simulink model "playback_data"  (R2015a)
settings: Solver=FixedStepDiscrete  SolverMode=SingleTasking  StartTime=76  StopTime=110  FixedStep=sample_time  RelTol=1e-3
undefined symbols (not defined in the file): A1_notch_f1, A2_notch_f1, A_kalman_swing_load, A_kalman_transverse, A_kalman_vertical, A_lpf_accelerometer, A_lpf_dtau, A_lpf_fourbar_angles, A_lpf_imu, A_lpf_lateral_angle, B1_lpf_accelerometer, B1_lpf_dtau, B1_lpf_fourbar_angles, B1_lpf_imu, B1_lpf_lateral_angle, B1_notch_f1, B2_lpf_accelerometer, B2_lpf_dtau, B2_lpf_fourbar_angles, B2_lpf_imu, B2_lpf_lateral_angle, B2_notch_f1, B_dx_versus_x0, B_kalman_swing_load, B_kalman_transverse, B_kalman_vertical, backwards_K_sag_of_t, backwards_P_sag_of_t, C_kalman_swing_load, C_kalman_transverse, C_kalman_vertical, com_leg_motor, com_torso, contact_threshold, control_start_time, d_ankle_to_foot, d_vertical_com, desired_com_forward_velocity, desired_com_lateral_velocity, desired_initial_leg_roll_left, desired_initial_leg_roll_right, desired_stance_beta2, desired_standing_torso_pitch, desired_standing_torso_roll, desired_standing_z, desired_torso_pitch, desired_torso_roll, Discrete, enable_bouncing, fcut_contact, fdesignblkfcn, forward_dx_of_dxstar, forward_x_of_dxstar, g, gcbh, HIP_MTR_MAX_CONT_TORQUE, HIP_MTR_MAX_TORQUE, i_leg_motor, i_robot, i_torso ... (+78)
libraries: simulink x65, dsparch4 x18, ctrlSharedLib x14, dspfdesign x4
(part 2 of 13)

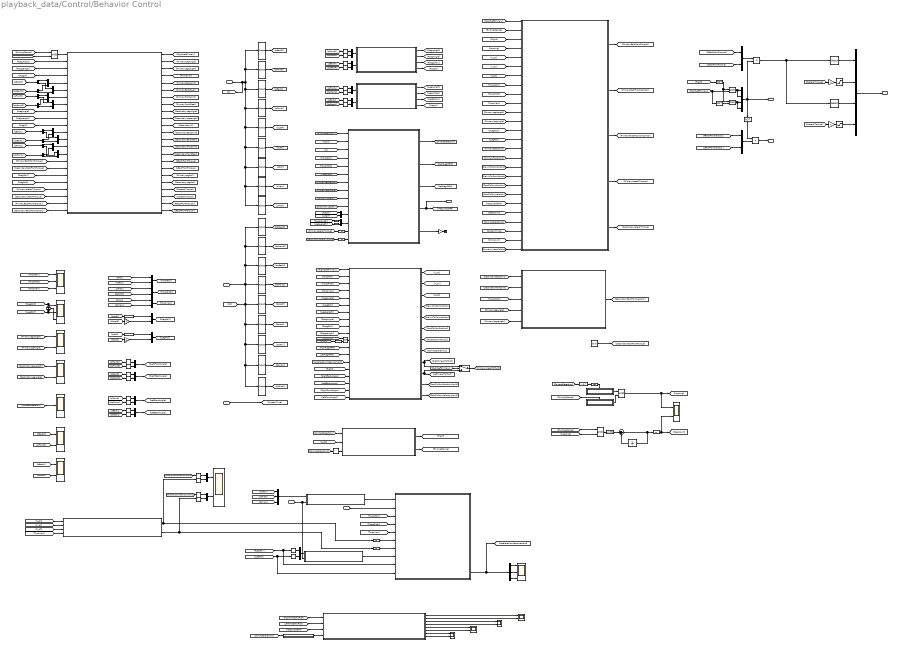
== system playback_data/Control/Behavior Control ==
  note: Signal Routing
  note: Begin Control
  note: Position & Velocity Estimation
  note: Force Estimation
  note: Leg/Spring Measurements
  note: Torque Commands
  note: Secondary Leg Behavior
  note: Primary Leg + Lateral Behavior
  note: Inputs
  note: q Order:
      |
      | backJointR
      | backGearR
      | frontJointR
      | frontGearR
      |
      | backJointL
      | backGearL
      | frontJointL
      | frontGearL
      |
      | latR
      | latL
      |
      | torsoRoll
      | torsoYaw
      | torsoPitch
  note: Motor Order:
      |
      | backR
      | frontR
      | latR
      | backL
      | frontL
      | latL
  note: Angle Conversions
  note: Contact Estimation
  note: Logging
  note: Acceleration Measurement
  note: Knee Torque Estimation
  Enabled [true/false] : Inport
  Body XYZ Acceleration [m/s^2] x3 : Inport  Port=2
  dq : Inport  Port=3
  q : Inport  Port=4
  time : Inport  Port=5
  At Least One Stance Detected : Subsystem
  COM Acceleration Measurement : Scope  NumInputPorts=3
      settings: YMin=-10~-12.5~-15  YMax=7.5~7.5~15  SaveName=ScopeData34  SampleInput=on
  COM World Frame X : Scope  NumInputPorts=2
      settings: TimeRange=3.175000000000004  YMin=-0.004~-0.175  YMax=0.02~0.225  SaveName=ScopeData35  SampleInput=on
  Compare To Constant : simulink/Logic and Bit Operations/Compare To Constant  relop=>  const=0.7  OutDataTypeStr=boolean
  Compute COM Translational Acceleration (IMU uses non-rotating measurement frame) : MATLAB Function  TreatAsAtomicUnit=on
  Compute Forces1 : Subsystem
  Compute World Frame COM Coordinates from Yawed Frame : MATLAB Function  TreatAsAtomicUnit=on
  Constant : Constant  Value=[0 0]
  Contact : Scope
      settings: YMin=0.3  YMax=0.9  SaveName=ScopeData11  SampleInput=on
  Contact State Machine : Subsystem
  Data Type Conversion : DataTypeConversion  OutDataTypeStr=uint32
  Demux : Demux  Outputs=3
  Demux{3..10} (8 alike) : Demux  Outputs=2
  Estimate Angular Accelerations2 : Subsystem
  Estimate Angular Accelerations3 : Subsystem
  Exited Stance : Subsystem
  Force Estimation : Subsystem
  Gain{1..2,12..13} (4 alike) : Gain  Gain=-1
  Hopping / Steps : Scope  NumInputPorts=2
      settings: YMin=1~1  YMax=1~1  SaveName=ScopeData33  SampleInput=on
  Knee Torques : MATLAB Function  TreatAsAtomicUnit=on
  L Knee Torques from Accelerometer : Scope  NumInputPorts=2
      settings: YMin=-1000~-1250  YMax=1500~2000  SaveName=ScopeData42  SampleInput=on
  L Knee Torques from Forward Dynamics : Scope  NumInputPorts=2
      settings: YMin=-75~-220  YMax=250~0  SaveName=ScopeData43  SampleInput=on
  L Leg Calculator : Subsystem
  Left Lateral Torque Saturation : Saturate  UpperLimit=max_torque_lateral  LowerLimit=-max_torque_lateral
      settings: AttributesFormatString=Top: %<UpperLimit>\nBottom: %<LowerLimit>
  Left Leg Fourbar Positions : Scope  NumInputPorts=2
      settings: YMin=4.05~2.275  YMax=4.17~2.375  SaveName=ScopeData17  SampleInput=on
  Logical Operator : Logic  IconShape=distinctive  AllPortsSameDT=off  OutDataTypeStr=boolean
  Logical Operator{1,3,5,7} (4 alike) : Logic  AllPortsSameDT=off  OutDataTypeStr=boolean
  Logical Operator2 : Logic  Operator=OR  AllPortsSameDT=off  OutDataTypeStr=boolean
  Logical Operator{4,6,8..9} (4 alike) : Logic  Operator=NOT  AllPortsSameDT=off  OutDataTypeStr=boolean
  Mux : Mux
  Mux{1..2,4..24,26..27,30..31,33} (28 alike) : Mux  Inputs=2
  Mux28 : Mux  Inputs=3
  Mux3 : Mux
  Primary Leg Length / Angle : Scope  NumInputPorts=2
      settings: YMin=0.3~0  YMax=0.9~3.5  SaveName=ScopeData21  SampleInput=on
  Primary Secondary Leg Swap : Subsystem
  Primary and Lateral Behavior : Subsystem
  Product : Product
  Product1 : Product
  R Knee Torques from Accelerometer : Scope  NumInputPorts=2
      settings: YMin=0.95~0.95  YMax=1.05~1.05  SaveName=ScopeData41  SampleInput=on
  R Knee Torques from Forward Dynamics : Scope  NumInputPorts=2
      settings: YMin=0.95~0.95  YMax=1.05~1.05  SaveName=ScopeData40  SampleInput=on
  R Leg Calculator : Subsystem
  Right Lateral Torque Saturation : Saturate  UpperLimit=max_torque_lateral  LowerLimit=-max_torque_lateral
      settings: AttributesFormatString=Top: %<UpperLimit>\nBottom: %<LowerLimit>
  Right Left Symmetry Leg Roll : Scope  NumInputPorts=3
      settings: YMin=-0.2~-0.5~-0.5  YMax=1.3~1.8~0.5  SaveName=ScopeData19  SampleInput=on
  Right Leg Fourbar Positions : Scope  NumInputPorts=2
      settings: YMin=3.19015~1.00606  YMax=3.99645~2.79375  SaveName=ScopeData16
  Roll Pitch Yaw : Scope  NumInputPorts=3
      settings: YMin=-1000~-5~-5  YMax=1000~5~5  SampleInput=on
  Secondary Leg Behavior : Subsystem
  Secondary Leg Length / Angle : Scope  NumInputPorts=2
      settings: YMin=-1~-0.8  YMax=1~1.4  SaveName=ScopeData22  SampleInput=on
  Selector : Selector  InputPortWidth=4  Indices=[1 2]
  Selector1 : Selector  InputPortWidth=13  Indices=[10]
  Selector10 : Selector  InputPortWidth=13  Indices=[7 8]
  Selector11 : Selector  InputPortWidth=13  Indices=[9]
  Selector12 : Selector  InputPortWidth=13  Indices=[1 2]
  Selector13 : Selector  InputPortWidth=13  Indices=[3 4]
  Selector{14..17,19,24..27,29..37} (18 alike) : Selector  InputPortWidth=2  Indices=[1]
  Selector18 : Selector  InputPortWidth=13  Indices=[13]
  Selector2 : Selector  InputPortWidth=13  Indices=[5 6]
  Selector20 : Selector  InputPortWidth=13  Indices=[13]
  Selector21 : Selector  InputPortWidth=13  Indices=[11]
  Selector22 : Selector  InputPortWidth=13  Indices=[12]
  Selector23 : Selector  InputPortWidth=13  Indices=[11]
  Selector28 : Selector  InputPortWidth=13  Indices=[12]
  Selector3 : Selector  InputPortWidth=4  Indices=[3 4]
  Selector38 : Selector  InputPortWidth=3  Indices=[3]
  Selector4 : Selector  InputPortWidth=13  Indices=[7 8]
  Selector41 : Selector  InputPortWidth=2  Indices=[2]
  Selector42 : Selector  InputPortWidth=2  Indices=[2]
  Selector{43..46} (4 alike) : Selector  InputPortWidth=3  Indices=[1]
  Selector5 : Selector  InputPortWidth=13  Indices=[9]
  Selector6 : Selector  InputPortWidth=13  Indices=[1 2]
  Selector7 : Selector  InputPortWidth=13  Indices=[3 4]
  Selector8 : Selector  InputPortWidth=13  Indices=[10]
  Selector9 : Selector  InputPortWidth=13  Indices=[5 6]
  State Estimation : Subsystem
  Sum1 : Sum  Inputs=|++  OutMin=0
  Sum3 : Sum  Inputs=-|+
  Switch : Switch  Criteria=u2 ~= 0
  Terminator6 : Terminator
  Unit Delay : UnitDelay  SampleTime=-1
  Unit Delay{1..6} (6 alike) : UnitDelay  SampleTime=sample_time
  lateral_coordinates : Fcn  Expr=pi/2-u
  lateral_coordinates1 : Fcn  Expr=pi/2-u
  torso_roll_acceleration : Gain
  Torque Commands [Nm] x6 : Outport  OutputWhenDisabled=reset  InitialOutput=[0 0 0 0 0 0]
  Velocity Commands [rad/s] x4 : Outport  Port=2  OutputWhenDisabled=reset  InitialOutput=[0 0 0 0 0 0]
  Stance / Swing Control [1/0] x4 : Outport  Port=3  OutputWhenDisabled=reset  InitialOutput=[0 0 0 0 0 0]
  GRF XYZ estimates [N N N] : Outport  Port=4  OutputWhenDisabled=reset  InitialOutput=[0 0 0 0 0 0]
  wires:
  Selector46/1 -> Mux33/1
  Selector45/1 -> Mux31/1
  Selector44/1 -> Mux31/2
  Selector43/1 -> Mux33/2
  [FootToComPositionWorld] -> Selector46/1
  [FootToComVelocityWorld] -> Selector45/1
  Mux31/1 -> COM World Frame X/2
  Mux33/1 -> COM World Frame X/1
  [TorsoYaw] -> Compute World Frame COM Coordinates from Yawed Frame/4(torso_yaw)
  [Z_dZ] -> Compute World Frame COM Coordinates from Yawed Frame/3(Z_dZ)
  [Y_dY] -> Compute World Frame COM Coordinates from Yawed Frame/2(Y_dY)
  [X_dX] -> Compute World Frame COM Coordinates from Yawed Frame/1(X_dX)
  Compute World Frame COM Coordinates from Yawed Frame/1(com_position_world) -> Selector43/1, Unit Delay5/1
  Compute World Frame COM Coordinates from Yawed Frame/2(com_velocity_world) -> Selector44/1, Unit Delay6/1
  Unit Delay6/1 -> Compute COM Translational Acceleration (IMU uses non-rotating measurement frame)/7(com_velocity_world)
  Unit Delay5/1 -> Compute COM Translational Acceleration (IMU uses non-rotating measurement frame)/6(com_position_world)
  [TorsoYaw] -> Compute COM Translational Acceleration (IMU uses non-rotating measurement frame)/5(torso_yaw)
  Estimate Angular Accelerations3/1(Angular Accelerations [rad/s^2] x2) -> Compute COM Translational Acceleration (IMU uses non-rotating measurement frame)/8(hip_roll_accelerations)
  Mux30/1 -> Estimate Angular Accelerations3/1(Angular Velocities [rad/s] x2)
  Selector42/1 -> Mux30/2
  Selector41/1 -> Mux30/1
  [LLegRoll] -> Compute COM Translational Acceleration (IMU uses non-rotating measurement frame)/10(left_hip_roll), Selector42/1
  [RLegRoll] -> Compute COM Translational Acceleration (IMU uses non-rotating measurement frame)/9(right_hip_roll), Selector41/1
  Estimate Angular Accelerations2/1(Angular Accelerations [rad/s^2] x3) -> Compute COM Translational Acceleration (IMU uses non-rotating measurement frame)/1(torso_angular_accelerations)
  Body XYZ Acceleration [m/s^2] x3/1 -> Compute COM Translational Acceleration (IMU uses non-rotating measurement frame)/2(imu_translational_accelerations_body)
  Enabled [true/false]/1 -> Estimate Angular Accelerations3/2(Enabled), Estimate Angular Accelerations2/2(Enabled)
  Mux28/1 -> Estimate Angular Accelerations2/1(Angular Velocities [rad/s] x3)
  [dqYaw] -> Mux28/3
  [dqPitch] -> Mux28/2
  [dqRoll] -> Mux28/1
  [TorsoRoll] -> Compute COM Translational Acceleration (IMU uses non-rotating measurement frame)/3(torso_roll)
  [TorsoPitch] -> Compute COM Translational Acceleration (IMU uses non-rotating measurement frame)/4(torso_pitch)
  Demux/3 -> COM Acceleration Measurement/3
  Demux/1 -> COM Acceleration Measurement/1
  Demux/2 -> COM Acceleration Measurement/2
  Compute COM Translational Acceleration (IMU uses non-rotating measurement frame)/6(com_acceleration_yawed) -> [AccelerationMeasurement], Demux/1
  Switch/1 -> [PrimaryKneesToFoot]
  [RightLeftPrimary] -> Switch/2
  [LeftFrontAngle] -> State Estimation/19(Left Front [rad rad/s])
  [RightFrontAngle] -> State Estimation/18(Right Front [rad rad/s])
  [LeftBackAngle] -> State Estimation/17(Left Back [rad rad/s])
  [RightBackAngle] -> State Estimation/16(Right Back [rad rad/s])
  State Estimation/10(Left Knees to Foot [m m m] x2) -> [LeftKneesToFoot], Switch/3
  State Estimation/9(Right Knees to Foot [m m m] x2) -> Switch/1, [RightKneesToFoot]
  State Estimation/8(COM Acceleration [m/s^2] x3) -> [ComAccelerations]
  [AccelerationMeasurement] -> State Estimation/14(" Acceleration Measurement [m/s^2] x3")
  State Estimation/1("Horizontal COM [m, m/s]") -> [X_dX]
  State Estimation/3("Vertical COM [m, m/s]") -> [Z_dZ]
  [RLegLength] -> State Estimation/10(Right Leg Length [m m/s])
  [TorsoRoll] -> State Estimation/2(Torso Roll [rad rad/s])
  [TorsoPitch] -> State Estimation/3(Torso Pitch [rad rad/s])
  [RLegRoll] -> State Estimation/9(Right Leg Roll [rad rad/s])
  [LLegRoll] -> State Estimation/6(Left Leg Roll [rad rad/s])
  [LLegLength] -> State Estimation/7(Left Leg Length [m m/s])
  [LLegAngle] -> State Estimation/5(Left Leg Sagittal Angle [rad rad/s])
  [RLegAngle] -> State Estimation/8(Right Leg Sagittal Angle [rad rad/s])
  [RightLeftPrimary] -> State Estimation/1(Right or Left [1/0])
  Logical Operator2/1 -> State Estimation/11(Enable Kalman Filtering [1/0])
  [RightLegGRFs] -> State Estimation/12(Right GRF [X Y Z] [N N N])
  [LeftLegGRFs] -> State Estimation/13(Left GRF [X Y Z] [N N N])
  State Estimation/4(Pelvis to COM Position [m m m]) -> [PelvisToComPosition]
  State Estimation/5(Pelvis to COM Velocity [m/s m/s m/s]) -> [PelvisToComVelocity]
  State Estimation/2("Lateral COM [m, m/s]") -> [Y_dY]
  [TorsoYaw] -> State Estimation/4(Torso Yaw [rad rad/s])
  State Estimation/6(Foot to COM Position [m m m]) -> [FootToComPosition]
  State Estimation/7(Foot to COM Velocity [m/s m/s m/s]) -> [FootToComVelocity]
  [hopping] -> Logical Operator2/1
  Logical Operator4/1 -> Logical Operator2/2
  [flight] -> Logical Operator4/1
  [flight] -> State Estimation/15(Flight [1/0])
  State Estimation/11(COM Position World [m m m]) -> [FootToComPositionWorld]
  State Estimation/12(COM Velocity World [m/s m/s m/s]) -> [FootToComVelocityWorld]
  [ExitingStance] -> Exited Stance/Enable
  Data Type Conversion/1 -> Sum1/1
  Logical Operator1/1 -> Data Type Conversion/1
  Sum1/1 -> Unit Delay/1, Unit Delay2/1
  Unit Delay/1 -> Sum1/2
  [RLateralTorque] -> Gain2/1
  [SecondaryBackJoint] -> Secondary Leg Behavior/1(Secondary Back Load [rad rad/s])
  [SecondaryFrontJoint] -> Secondary Leg Behavior/2(Secondary Front Load [rad rad/s])
  Primary and Lateral Behavior/3(Primary Force or Position Control [1/0]) -> [PrimaryForcePositionControl]
  Primary and Lateral Behavior/1(Primary Back/Front SEA Torques [Nm] x2) -> [PrimaryBackFrontTorque]
  Primary Secondary Leg Swap/1(Right/Left Primary [1/0]) -> [RightLeftPrimary]
  Logical Operator/1 -> Primary Secondary Leg Swap/1(Exiting Stance [1/0])
  Primary Secondary Leg Swap/17(L Back/Front SEA Torque [Nm Nm]) -> [LBackFrontTorque]
  Primary Secondary Leg Swap/16(R Back/Front SEA Torque [Nm Nm]) -> [RBackFrontTorque]
  Primary Secondary Leg Swap/11(Secondary Leg w [m]) -> [SecondaryW]
  Primary Secondary Leg Swap/15(Secondary Front Gear [rad rad/s]) -> [SecondaryFrontGear]
  Primary Secondary Leg Swap/14(Secondary Front Joint [rad rad/s]) -> [SecondaryFrontJoint]
  Primary Secondary Leg Swap/13(Secondary Back Gear [rad rad/s]) -> [SecondaryBackGear]
  Primary Secondary Leg Swap/12(Secondary Back Joint [rad rad/s]) -> [SecondaryBackJoint]
  Primary Secondary Leg Swap/8(Primary Front Gear [rad rad/s]) -> [PrimaryFrontGear]
  Primary Secondary Leg Swap/7(Primary Front Joint [rad rad/s]) -> [PrimaryFrontJoint]
  Primary Secondary Leg Swap/6(Primary Back Gear [rad rad/s]) -> [PrimaryBackGear]
  Primary Secondary Leg Swap/5(Primary Back Joint [rad rad/s]) -> [PrimaryBackJoint]
  [SecondaryBackFrontTorque] -> Primary Secondary Leg Swap/17(Secondary Back/Front SEA Torque [Nm Nm])
  [PrimaryBackFrontTorque] -> Primary Secondary Leg Swap/16(Primary Back/Front SEA Torque [Nm Nm])
  Demux9/2 -> Mux13/2
  Demux9/1 -> Mux16/2
  Demux10/2 -> Mux13/1
  Demux10/1 -> Mux16/1
  [qBackL] -> Demux10/1
  [dqBackL] -> Demux9/1
  Demux8/2 -> Mux15/2
  Demux8/1 -> Mux14/2
  Demux7/2 -> Mux15/1
  Demux7/1 -> Mux14/1
  Mux15/1 -> Primary Secondary Leg Swap/15(L Front Gear [rad rad/s])
  Mux14/1 -> Primary Secondary Leg Swap/14(L Front Joint [rad rad/s])
  Mux13/1 -> Primary Secondary Leg Swap/13(L Back Gear [rad rad/s])
  Mux16/1 -> Primary Secondary Leg Swap/12(L Back Joint [rad rad/s])
  [dqFrontL] -> Demux8/1
  [qFrontL] -> Demux7/1
  Demux5/2 -> Mux10/2
  Demux5/1 -> Mux9/2
  Demux6/2 -> Mux10/1
  Demux6/1 -> Mux9/1
  [qBackR] -> Demux6/1
  [dqBackR] -> Demux5/1
  Demux4/2 -> Mux12/2
  Demux4/1 -> Mux11/2
  Demux3/2 -> Mux12/1
  Demux3/1 -> Mux11/1
  Mux12/1 -> Primary Secondary Leg Swap/8(R Front Gear [rad rad/s])
  Mux11/1 -> Primary Secondary Leg Swap/7(R Front Joint [rad rad/s])
  Mux10/1 -> Primary Secondary Leg Swap/6(R Back Gear [rad rad/s])
  Mux9/1 -> Primary Secondary Leg Swap/5(R Back Joint [rad rad/s])
  [dqFrontR] -> Demux4/1
  [qFrontR] -> Demux3/1
  Primary Secondary Leg Swap/9(Secondary Leg Angle [rad rad/s]) -> [SecondaryLegAngle]
  Primary Secondary Leg Swap/10(Secondary Leg Length [rad rad/s]) -> [SecondaryLegLength]
  [LLegW] -> Primary Secondary Leg Swap/11(L Leg w [m])
  [LLegLength] -> Primary Secondary Leg Swap/10(L Leg Length [m m/s])
  [LLegAngle] -> Primary Secondary Leg Swap/9(L Leg Angle [rad rad/s])
  [RLegW] -> Primary Secondary Leg Swap/4(R Leg w [m])
  [RLegLength] -> Primary Secondary Leg Swap/3(R Leg Length [m m/s])
  [RLegAngle] -> Primary Secondary Leg Swap/2(R Leg Angle [rad rad/s])
  Primary Secondary Leg Swap/3(Primary Leg Length [m m/s]) -> [PrimaryLegLength]
  Primary Secondary Leg Swap/4(Primary Leg w [m]) -> [PrimaryW]
  Primary Secondary Leg Swap/2(Primary Leg Angle [rad rad/s]) -> [PrimaryLegAngle]
  [TorsoPitch] -> Secondary Leg Behavior/3(Torso Pitch [rad rad/s])
  L Leg Calculator/4(w [m]) -> [LLegW]
  R Leg Calculator/4(w [m]) -> [RLegW]
  Selector26/1 -> Mux4/1
  Selector27/1 -> Mux4/2
  Selector25/1 -> Mux5/2
  Selector24/1 -> Mux5/1
  L Leg Calculator/3(Leg Splay [rad rad/s]) -> [LLegSplay]
  L Leg Calculator/2(Leg Angle [rad rad/s]) -> [LLegAngle]
  L Leg Calculator/1("Leg Length [m m/s] ") -> [LLegLength]
  Mux4/1 -> L Leg Calculator/2(Back [rad rad/s])
  Mux5/1 -> L Leg Calculator/1(Front [rad rad/s])
  [dqFrontL] -> Selector25/1
  [qFrontL] -> Selector24/1
  [dqBackL] -> Selector27/1
  [qBackL] -> Selector26/1
  Selector23/1 -> [qRoll]
  Selector18/1 -> [qPitch]
  q/1 -> [q], Selector1/1, Selector23/1, Selector28/1, Selector18/1, Selector5/1, Selector4/1, Selector2/1, Selector7/1, Selector6/1
  Selector16/1 -> Mux1/1
  Selector17/1 -> Mux1/2
  Selector15/1 -> Mux2/2
  Selector14/1 -> Mux2/1
  R Leg Calculator/3(Leg Splay [rad rad/s]) -> [RLegSplay]
  R Leg Calculator/2(Leg Angle [rad rad/s]) -> [RLegAngle]
  R Leg Calculator/1("Leg Length [m m/s] ") -> [RLegLength]
  Mux1/1 -> R Leg Calculator/2(Back [rad rad/s])
  Mux2/1 -> R Leg Calculator/1(Front [rad rad/s])
  [dqFrontR] -> Selector15/1
  [qFrontR] -> Selector14/1
  [dqBackR] -> Selector17/1
  [qBackR] -> Selector16/1
  Selector5/1 -> [qLatR]
  Selector1/1 -> [qLatL]
  Selector6/1 -> [qBackR]
  Selector7/1 -> [qFrontR]
  Selector2/1 -> [qBackL]
  Selector4/1 -> [qFrontL]
  [PrimaryLegAngle] -> Secondary Leg Behavior/4(Primary Leg Angle [rad rad/s])
  [PrimaryLegLength] -> Secondary Leg Behavior/5(Primary Leg Length [m m/s])
  Selector28/1 -> [qYaw]
  Force Estimation/1(Leg Plane Force for Contact Detection [body weight]) -> [ContactDetection]
  Force Estimation/2(Right GRF [X Y Z] [N N N]) -> [RightLegGRFs]
  [LLateralTorque] -> Gain1/1
  Force Estimation/3(Left GRF [X Y Z] [N N N]) -> [LeftLegGRFs]
  Force Estimation/4(GRF XYZ estimates [N N N]) -> GRF XYZ estimates [N N N]/1, [MeasuredGRF]
  Primary Secondary Leg Swap/18("Primary Leg Roll [rad, rad/s]") -> [PrimaryLegRoll]
  Primary Secondary Leg Swap/19("Secondary Leg Roll [rad, rad/s]") -> [SecondaryLegRoll]
  [RLegRoll] -> Primary Secondary Leg Swap/18("Right Leg Roll [rad, rad/s]")
  [LLegRoll] -> Primary Secondary Leg Swap/19("Left Leg Roll [rad, rad/s]")
  Unit Delay2/1 -> Hopping / Steps/2, [StepCount]
  [ExitingStance] -> Logical Operator1/1
  [hopping] -> Logical Operator1/2
  [hopping] -> Logical Operator/2
  [ExitingStance] -> Logical Operator/1
  [RightLeftPrimary] -> Force Estimation/1(Right/Left Primary)
  [flight] -> Force Estimation/2(Flight [1/0])
  [TorsoRoll] -> Force Estimation/4(Torso Roll [rad rad/s])
  [TorsoYaw] -> Force Estimation/6(Torso Yaw [rad rad/s])
  [TorsoPitch] -> Force Estimation/5(Torso Pitch [rad rad/s])
  [q] -> Force Estimation/3(q)
  [PrimaryLegLength] -> Force Estimation/7(Primary Leg Length [m m/s])
  [PrimaryLegAngle] -> Force Estimation/8(Primary Leg Angle [rad rad/s])
  [PrimaryLegRoll] -> Force Estimation/9(Primary Leg Roll [rad rad/s])
  [RLegW] -> Mux19/1
  [LLegW] -> Mux19/2
  Mux19/1 -> Force Estimation/11(Leg Width Right/Left [m m])
  [RLegLength] -> Selector19/1
  Mux20/1 -> Force Estimation/12(Leg Length Right/Left [m m])
  [SecondaryLegRoll] -> Force Estimation/10(Secondary Leg Roll [rad rad/s])
  [PrimaryLateralTorque] -> Unit Delay3/1
  [SecondaryLateralTorque] -> Unit Delay4/1
  torso_roll_acceleration/1 -> Terminator6/1
  Force Estimation/5(Torso Roll Acceleration [rad/s^2]) -> torso_roll_acceleration/1
  [PrimaryLateralTorque] -> Primary Secondary Leg Swap/20(Primary Lateral Torque [Nm])
  [SecondaryLateralTorque] -> Primary Secondary Leg Swap/21(Secondary Lateral Torque [Nm])
  Primary Secondary Leg Swap/20(Right Lateral Torque [Nm]) -> [RLateralTorque]
  Primary Secondary Leg Swap/21(Left Lateral Torque [Nm]) -> [LLateralTorque]
  Right Lateral Torque Saturation/1 -> Mux/2
  Left Lateral Torque Saturation/1 -> Mux/4
  Primary and Lateral Behavior/5(Secondary Lateral Torque [Nm]) -> [SecondaryLateralTorque]
  Primary and Lateral Behavior/4(Primary Lateral Torque [Nm]) -> [PrimaryLateralTorque]
  Selector19/1 -> Mux20/1
  [LLegLength] -> Selector29/1
  Selector29/1 -> Mux20/2
  Unit Delay3/1 -> Force Estimation/13(Primary Lateral Torque [Nm])
  Unit Delay4/1 -> Force Estimation/14(Secondary Lateral Torque [Nm])
  Logical Operator3/1 -> Hopping / Steps/1, [hopping]
  Gain2/1 -> Right Lateral Torque Saturation/1
  Gain1/1 -> Left Lateral Torque Saturation/1
  [TorsoYaw] -> Primary and Lateral Behavior/10(Torso Yaw [rad rad/s])
  [LLegRoll] -> Primary and Lateral Behavior/14(Left Leg Roll [rad rad/s])
  [RLegRoll] -> Primary and Lateral Behavior/13(Right Leg Roll [rad rad/s])
  [Y_dY] -> Primary and Lateral Behavior/6("[y,  dy] [m, m/s]")
  [StepCount] -> Primary and Lateral Behavior/22(Steps Taken)
  [MeasuredGRF] -> Primary and Lateral Behavior/21(Measured GRF [N N N])
  [TorsoRoll] -> Primary and Lateral Behavior/8(Torso Roll [rad rad/s])
  [Z_dZ] -> Primary and Lateral Behavior/7("[z, dz] [m, m/s]")
  [X_dX] -> Primary and Lateral Behavior/5("[x, dx] [m, m/s]")
  [PelvisToComVelocity] -> Primary and Lateral Behavior/18(Pelvis to COM Velocity [m m m])
  [PelvisToComPosition] -> Primary and Lateral Behavior/17(Pelvis to COM Position [m m m])
  [TorsoPitch] -> Primary and Lateral Behavior/9(Torso Pitch [rad rad/s])
  [PrimaryFrontJoint] -> Primary and Lateral Behavior/16(Primary Front Load [rad rad/s])
  [PrimaryLegLength] -> Primary and Lateral Behavior/11(Leg Length [m m/s])
  [hopping] -> Primary and Lateral Behavior/4(Hopping [1/0])
  [RightLeftPrimary] -> Primary and Lateral Behavior/1(Right/Left [1/0])
  [PrimaryBackJoint] -> Primary and Lateral Behavior/15(Primary Back Load [rad rad/s])
  [PrimaryLegAngle] -> Primary and Lateral Behavior/12(Leg Angle [rad rad/s])
  Contact State Machine/1(flight [1/0]) -> [flight]
  [FootToComVelocity] -> Primary and Lateral Behavior/20(Foot to COM Velocity [m m m])
  [FootToComPosition] -> Primary and Lateral Behavior/19(Foot to COM Position [m m m])
  Contact State Machine/2(Exiting Stance [1/0]) -> [ExitingStance]
  [flight] -> Primary and Lateral Behavior/3(Flight [1/0])
  [ContactDetection] -> Contact State Machine/1(Contact Factor [body weight])
  [Z_dZ] -> Contact State Machine/2("[Z dZ] [m m/s]")
  [ExitingStance] -> Primary and Lateral Behavior/2(Exiting Stance [1/0])
  [TorsoYaw] -> Roll Pitch Yaw/3
  [TorsoPitch] -> Roll Pitch Yaw/2
  [TorsoRoll] -> Roll Pitch Yaw/1
  [LLegRoll] -> Sum3/2, Right Left Symmetry Leg Roll/2
  [RLegRoll] -> Sum3/1, Right Left Symmetry Leg Roll/1
  Sum3/1 -> Right Left Symmetry Leg Roll/3
  [PrimaryLegLength] -> Primary Leg Length / Angle/1
  [PrimaryLegAngle] -> Primary Leg Length / Angle/2
  [SecondaryLegLength] -> Secondary Leg Length / Angle/1
  [SecondaryLegAngle] -> Secondary Leg Length / Angle/2
  [ContactDetection] -> Contact/1
  Secondary Leg Behavior/1(Secondary Back/Front Motor Torque [Nm Nm]) -> [SecondaryBackFrontVelocity]
  Mux21/1 -> [TorsoYaw]
  Mux23/1 -> [TorsoRoll]
  Mux7/1 -> [TorsoPitch]
  [dqRoll] -> Mux23/2
  [dqPitch] -> Mux7/2
  [qLatR] -> lateral_coordinates/1
  [dqLatR] -> Gain12/1
  [qLatL] -> lateral_coordinates1/1
  [dqLatL] -> Gain13/1
  Mux22/1 -> [RLegRoll]
  Mux24/1 -> [LLegRoll]
  lateral_coordinates/1 -> Mux22/1
  lateral_coordinates1/1 -> Mux24/1
  Gain13/1 -> Mux24/2
  Gain12/1 -> Mux22/2
  Selector8/1 -> [dqLatL]
  Selector11/1 -> [dqLatR]
  Selector12/1 -> [dqBackR]
  Selector13/1 -> [dqFrontR]
  Selector9/1 -> [dqBackL]
  Selector10/1 -> [dqFrontL]
  Selector20/1 -> [dqPitch]
  Selector22/1 -> [dqYaw]
  Selector21/1 -> [dqRoll]
  dq/1 -> Selector10/1, [dq], Selector11/1, Selector21/1, Selector20/1, Selector22/1, Selector8/1, Selector12/1, Selector13/1, Selector9/1
  [qRoll] -> Mux23/1
  [qPitch] -> Mux7/1
  [qYaw] -> Mux21/1
  [dqYaw] -> Mux21/2
  [qBackR] -> Right Leg Fourbar Positions/1
  [qFrontR] -> Right Leg Fourbar Positions/2
  [qBackL] -> Left Leg Fourbar Positions/1
  [qFrontL] -> Left Leg Fourbar Positions/2
  [ComAccelerations] -> Primary and Lateral Behavior/23(COM XYZ Acceleration [m/s^2] x3)
  time/1 -> [SystemTime]
  [SystemTime] -> Primary and Lateral Behavior/24(System Time [s])
  [flight] -> Logical Operator6/1
  Logical Operator5/1 -> Mux3/2, Mux3/1
  Logical Operator6/1 -> Logical Operator7/1, Logical Operator5/1
  Logical Operator7/1 -> Mux3/4, Mux3/3
  Logical Operator8/1 -> Logical Operator7/2
  [RightLeftPrimary] -> Logical Operator8/1, Logical Operator5/2
  [PrimaryW] -> Primary and Lateral Behavior/25(Primary Leg Width [m])
  Selector/1 -> Mux/1
  Selector3/1 -> Mux/3
  Mux/1 -> Torque Commands [Nm] x6/1
  Mux3/1 -> Logical Operator9/1, Product1/2, Stance / Swing Control [1/0] x4/1
  [ContactDetection] -> Compare To Constant/1
  Compare To Constant/1 -> Unit Delay1/1
  At Least One Stance Detected/1(Stance?) -> Logical Operator3/1
  Exited Stance/1(Takeoff?) -> Logical Operator3/2
  Unit Delay1/1 -> At Least One Stance Detected/Enable
  Mux6/1 -> Product/2
  [RBackFrontVelocity] -> Mux6/1
  [LBackFrontVelocity] -> Mux6/2
  [PrimaryBackFrontVelocity] -> Primary Secondary Leg Swap/22(Primary Front/Back Velocity [rad/s rad/s])
  [SecondaryBackFrontVelocity] -> Primary Secondary Leg Swap/23(Secondary Front/Back Velocity [rad/s rad/s])
  Primary Secondary Leg Swap/22(Right Front/Back Velocity [rad/s rad/s]) -> [RBackFrontVelocity]
  Primary Secondary Leg Swap/23(Left Front/Back Velocity [rad/s rad/s]) -> [LBackFrontVelocity]
  Primary and Lateral Behavior/2(Primary Back/Front Gear Velocities [rad/s] x2) -> [PrimaryBackFrontVelocity]
  Product/1 -> Velocity Commands [rad/s] x4/1
  Logical Operator9/1 -> Product/1
  [RBackFrontTorque] -> Mux8/1
  [LBackFrontTorque] -> Mux8/2
  Mux8/1 -> Product1/1
  Product1/1 -> Selector3/1, Selector/1
  Constant/1 -> [SecondaryBackFrontTorque]
  [ComAccelerations] -> Compute Forces1/1(XYZ Acceleration)
  [RightKneesToFoot] -> Knee Torques/1(right_knees_to_foot)
  [LeftKneesToFoot] -> Knee Torques/2(left_knees_to_foot)
  [MeasuredGRF] -> Knee Torques/3(grf_from_seas)
  Compute Forces1/1(XYZ Force) -> Knee Torques/4(grf_from_accelerometer)
  Knee Torques/1(right_front_knee_torques_from_fd) -> R Knee Torques from Forward Dynamics/1
  Knee Torques/2(right_back_knee_torques_from_fd) -> R Knee Torques from Forward Dynamics/2
  Knee Torques/3(right_front_knee_torques_from_accelerometer) -> R Knee Torques from Accelerometer/1
  Knee Torques/4(right_back_knee_torques_from_accelerometer) -> R Knee Torques from Accelerometer/2
  Knee Torques/5(left_front_knee_torques_from_fd) -> L Knee Torques from Forward Dynamics/1
  Knee Torques/6(left_back_knee_torques_from_fd) -> L Knee Torques from Forward Dynamics/2
  Knee Torques/8(left_back_knee_torques_from_accelerometer) -> L Knee Torques from Accelerometer/2
  Knee Torques/7(left_front_knee_torques_from_accelerometer) -> L Knee Torques from Accelerometer/1
  [qBackR] -> Selector32/1
  [dqBackR] -> Selector33/1
  [qFrontR] -> Selector30/1
  [dqFrontR] -> Selector31/1
  Selector30/1 -> Mux18/1
  Selector31/1 -> Mux18/2
  Selector33/1 -> Mux17/2
  Selector32/1 -> Mux17/1
  [qBackL] -> Selector36/1
  [dqBackL] -> Selector37/1
  [qFrontL] -> Selector34/1
  [dqFrontL] -> Selector35/1
  Selector34/1 -> Mux27/1
  Selector35/1 -> Mux27/2
  Selector37/1 -> Mux26/2
  Selector36/1 -> Mux26/1
  Mux18/1 -> [RightFrontAngle]
  Mux17/1 -> [RightBackAngle]
  Mux27/1 -> [LeftFrontAngle]
  Mux26/1 -> [LeftBackAngle]
  [ComAccelerations] -> Selector38/1
  Selector38/1 -> Contact State Machine/3(ddZ [m/s^2])
  [PrimaryKneesToFoot] -> Primary and Lateral Behavior/26(Primary Knees to Foot [m] x6)

== system playback_data/Control/Compute Body Frame Accelerations ==
  accelerometer [g] x3 : Inport
  Convert to Body Frame IMU Accelerations : MATLAB Function  TreatAsAtomicUnit=on
  IMU Two Pole Filter2 : DiscreteTransferFcn  Numerator=[A_lpf_accelerometer 0 0]  Denominator=[1 B1_lpf_accelerometer B2_lpf_accelerometer]  InitialStates=[0, 0, g; 0, 0, g]*15.277  SampleTime=sample_time
  IMU XYZ Accelerations : Scope
      settings: YMin=-4  YMax=14  SaveName=ScopeData28  SampleInput=on
  Mux : Mux  Inputs=2
  accelerations [m/s^2] x3 : Outport
  wires:
  IMU Two Pole Filter2/1 -> accelerations [m/s^2] x3/1, Mux/2
  Mux/1 -> IMU XYZ Accelerations/1
  Convert to Body Frame IMU Accelerations/1(imu_accelerations) -> IMU Two Pole Filter2/1, Mux/1
  accelerometer [g] x3/1 -> Convert to Body Frame IMU Accelerations/1(accelerometer)

== system playback_data/Control/Filter Velocities ==
  raw dq : Inport
  Demux : Demux  Outputs=3
  Demux1 : Demux  Outputs=3
  Demux2 : Demux  Outputs=2
  Demux3 : Demux  Outputs=2
  Fourbar : Selector  InputPortWidth=13  Indices=[1 2 3 4 5 6 7 8]
  Fourbar Velocity Filter : Scope  NumInputPorts=4
      settings: YMin=-0.55~-0.4~-0.4~-0.6  YMax=0.25~0.7~0.45~0.5  SaveName=ScopeData14  SampleInput=on
  IMU Two Pole Filter : DiscreteTransferFcn  Numerator=[A_lpf_imu 0 0]  Denominator=[1 B1_lpf_imu B2_lpf_imu]  SampleTime=sample_time
  Lateral : Selector  InputPortWidth=13  Indices=[9 10]
  Lateral Angle Two Pole Filter1 : DiscreteTransferFcn  Numerator=[A_lpf_lateral_angle 0 0]  Denominator=[1 B1_lpf_lateral_angle B2_lpf_lateral_angle]  SampleTime=sample_time
  Lateral Angle Two Pole Filter2 : DiscreteTransferFcn  Numerator=[A_lpf_fourbar_angles 0 0]  Denominator=[1 B1_lpf_fourbar_angles B2_lpf_fourbar_angles]  SampleTime=sample_time
  Leg Roll Velocity Filter : Scope  NumInputPorts=2
      settings: YMin=-0.225~-1.5  YMax=0.175~2.25  SaveName=LegRollFilter  SampleInput=on
  Mux : Mux  Inputs=3
  Mux{25..33} (9 alike) : Mux  Inputs=2
  Selector1 : Selector  InputPortWidth=8  Indices=[1 2]
  Selector2 : Selector  InputPortWidth=8  Indices=[3 4]
  Selector3 : Selector  InputPortWidth=8  Indices=[5 6]
  Selector34 : Selector  InputPortWidth=8  Indices=[1 2]
  Selector35 : Selector  InputPortWidth=8  Indices=[3 4]
  Selector36 : Selector  InputPortWidth=8  Indices=[5 6]
  Selector37 : Selector  InputPortWidth=8  Indices=[7 8]
  Selector4 : Selector  InputPortWidth=8  Indices=[7 8]
  Torso Orientation : Selector  InputPortWidth=13  Indices=[11 12 13]
  Torso Orientation Filter : Scope  NumInputPorts=3
      settings: YMin=-0.2~-0.03~-0.15  YMax=0.125~0.0275~0.15  SaveName=ScopeData13  SampleInput=on
  filtered dq : Outport
  wires:
  Lateral Angle Two Pole Filter2/1 -> Selector4/1, Selector3/1, Selector2/1, Selector1/1, Mux/1
  IMU Two Pole Filter/1 -> Demux1/1, Mux/3
  Mux/1 -> filtered dq/1
  raw dq/1 -> Fourbar/1, Torso Orientation/1, Lateral/1
  Lateral/1 -> Demux2/1, Lateral Angle Two Pole Filter1/1
  Torso Orientation/1 -> IMU Two Pole Filter/1, Demux/1
  Lateral Angle Two Pole Filter1/1 -> Demux3/1, Mux/2
  Mux25/1 -> Torso Orientation Filter/1
  Mux27/1 -> Torso Orientation Filter/3
  Mux26/1 -> Torso Orientation Filter/2
  Mux30/1 -> Fourbar Velocity Filter/1
  Mux32/1 -> Fourbar Velocity Filter/3
  Mux31/1 -> Fourbar Velocity Filter/2
  Mux33/1 -> Fourbar Velocity Filter/4
  Selector34/1 -> Mux30/1
  Fourbar/1 -> Selector34/1, Selector35/1, Selector36/1, Selector37/1, Lateral Angle Two Pole Filter2/1
  Selector35/1 -> Mux31/1
  Selector36/1 -> Mux32/1
  Selector37/1 -> Mux33/1
  Mux28/1 -> Leg Roll Velocity Filter/1
  Mux29/1 -> Leg Roll Velocity Filter/2
  Demux/1 -> Mux25/1
  Demux/2 -> Mux26/1
  Demux/3 -> Mux27/1
  Demux1/1 -> Mux25/2
  Demux1/2 -> Mux26/2
  Demux1/3 -> Mux27/2
  Demux2/2 -> Mux29/1
  Demux2/1 -> Mux28/1
  Demux3/1 -> Mux28/2
  Demux3/2 -> Mux29/2
  Selector4/1 -> Mux33/2
  Selector3/1 -> Mux32/2
  Selector2/1 -> Mux31/2
  Selector1/1 -> Mux30/2
